simulink model "h175_model_cathode_Harness_HCTRL"  (R2023a)
settings: Solver=VariableStepAuto  StartTime=0.0  StopTime=4750  RelTol=1e-2
InitFcn:
  | run("cathode_subsystem_parameters.m")
undefined symbols (not defined in the file or in its folder): AIRCL_STATE, AIRCL_STATE_SAFETY, CSEP_STATE, CSEP_STATE_SAFETY, CSTOBLV_STATE_SAFETY, EAC_STATE, EAC_STATE_SAFETY, init_Parameters, sigbuilder_block, struct_OMM_Set, struct_Sensors
libraries: simulink x7, fl_lib x6, nesl_utility x6
settings Model: Creator=adrian.taveras  LastModifiedBy=adrian.taveras
settings SolverCC: MaxConsecutiveMinStep=20  ZeroCrossAlgorithm=Adaptive  DecoupledContinuousIntegration=on
settings DataIOCC: Refine=2
settings OptimizationCC: ReuseModelBlockBuffer=off
settings DebuggingCC: IgnoredZcDiagnostic=none
settings SimscapeCC: SimscapeLogType=all

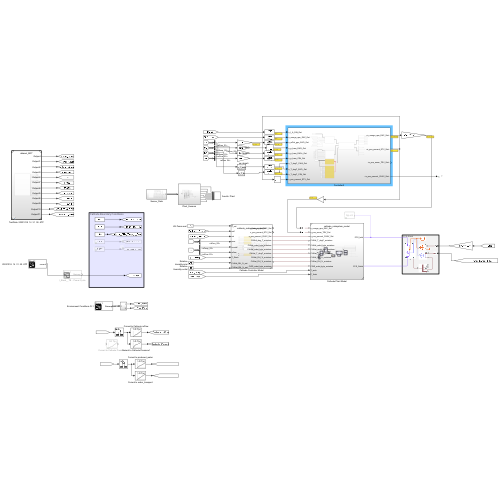
[thumbnail: Simulink's stored preview of the top-level diagram]
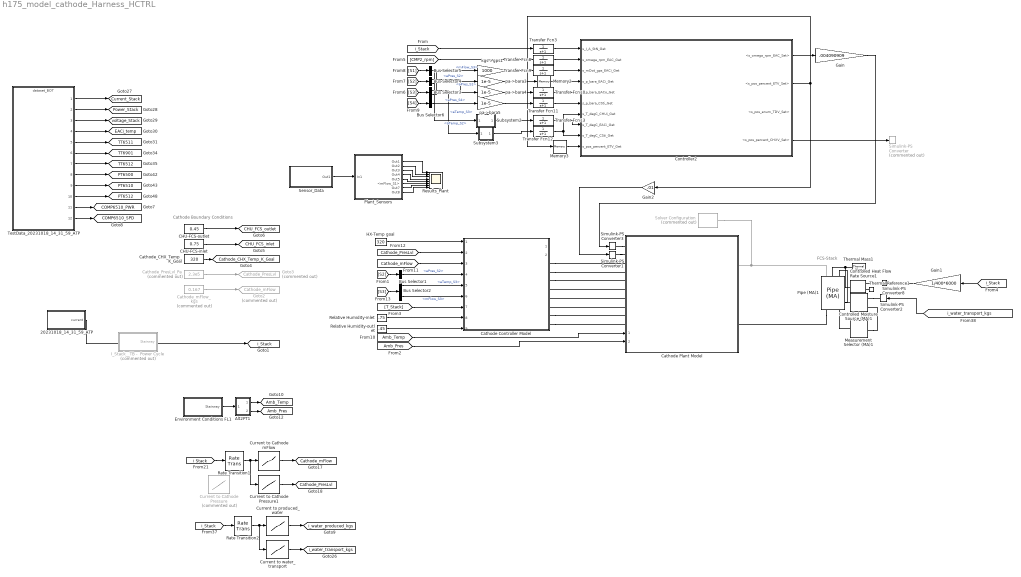
== system h175_model_cathode_Harness_HCTRL ==
  note: Cathode Boundary Conditions
  note: FCS-Stack
  20231018_14_31_59_ATP : Subsystem  Tag=STV Subsys  LoadFcn=sigbuilder_block('load');  StartFcn=sigbuilder_block('start');  StopFcn=sigbuilder_block('stop');  ClipboardFcn=sigbuilder_block('clipboard');  mask(Sigbuilder block){tuvar=[0:10]}
      mask help: Simulink:masks:SigbuilderBlock_MD
      mask init:
      | if ~strcmp(get_param(bdroot(gcbh),'SimulationStatus'),'stopped') tuvar = sigbuilder_block('maskInit'); end
      settings: CopyFcn=sigbuilder_block('copy');  DeleteFcn=sigbuilder_block('delete');  ModelCloseFcn=sigbuilder_block('modelClose');  PreSaveFcn=sigbuilder_block('preSave');  PauseFcn=sigbuilder_block('pause');  ContinueFcn=sigbuilder_block('continue');  NameChangeFcn=sigbuilder_block('namechange');  OpenFcn=sigbuilder_block('open',[725.25 330.75 938.25 556.5 ]);  CloseFcn=sigbuilder_block('close');
      mask Display: plot(0, 0, 100, 100,[2, 2, 32, 32, 2], [68, 8, 8, 68, 68],[32, 2], [38, 38], [32, 19, 2],[53, 60, 44], [32, 17, 17, 2],[16, 16, 31, 31]);txt = getActiveGroup(gcbh);text(2, 100, txt,'verticalAlignment', 'top');
  Alt2PT1 : Subsystem
  Bus Selector1 : BusSelector  OutputSignals=aPres_S2
  Bus Selector2 : BusSelector  OutputSignals=aTemp_S3,mFlow_S3
  Bus Selector3 : BusSelector  OutputSignals=aTemp_S3,mFlow_S3
  Bus Selector4 : BusSelector  OutputSignals=aPres_S2,aTemp_S2
  Bus Selector5 : BusSelector  OutputSignals=aPres_S1
  Bus Selector6 : BusSelector  OutputSignals=aPres_S4
  CHU-FCS-inlet : Constant  Value=0.75
  CHU-FCS-outlet : Constant  Value=0.45
  Cathode Controller Model : Subsystem  ReferencedSubsystem=cathode_subsystem_controller
      settings: PortSchema="{\"entries\":[{\"content\":{\"sides\":[{\"content\":{\"connectorIds\":[\"Out1\",\"Out2\",\"LConn1\",\"LConn2\",\"LConn3\",\"LConn4\",\"LConn5\",\"LConn6\",\"LConn7\",\"LConn8\"]},\"type\":\"ConnectorPlacement.EquallySpacedRectSide\",\"uuid\":\"fec6d33c-3ad3-4174-acdc-3a3b9e5715f4\"},{\"content\":{\"connectorIds\":[\"In1\",\"In2\",\"In3\",\"In4\",\"In5\",\"In6\",\"In7\",\"In8\",\"In9\"],\"side\":\"RIGHT\"},\"type\":\"ConnectorPlacement.EquallySpacedRectSide\",\"uuid\":\"4aee90de-c0ab-447d-83f7-53a254285efe\"},{\"content\":{\"side\":\"TOP\"},\"type\":\"ConnectorPlacement.EquallySpacedRectSide\",\"uuid\":\"94b2adb1-5e3a-4413-84ea-fe1e13b8a59d\"}]},\"type\":\"ConnectorPlacement.EquallySpacedConnector\",\"uuid\":\"aca8449a-2e64-4d0b-80a0-10fe30b1ea20\"}],\"packageUris\":[\"http://schema.mathworks.com/mf0/Connector/R2020b\"],\"version\":\"1.0\"}"
  Cathode Plant Model : Subsystem  ReferencedSubsystem=cathode_subsystem_model
      settings: PortSchema="{\"entries\":[{\"content\":{\"sides\":[{\"content\":{\"connectorIds\":[\"LConn10\",\"LConn9\",\"LConn1\",\"LConn2\",\"LConn3\",\"LConn4\",\"LConn5\",\"LConn6\",\"LConn7\",\"LConn8\",\"In1\",\"In2\"]},\"type\":\"ConnectorPlacement.EquallySpacedRectSide\",\"uuid\":\"e3b30cb5-20d3-4977-927f-9fea068a9234\"},{\"content\":{\"connectorIds\":[\"RConn1\",\"RConn2\"],\"side\":\"RIGHT\"},\"type\":\"ConnectorPlacement.EquallySpacedRectSide\",\"uuid\":\"2d547627-9665-492a-afa4-fcc16b1173a1\"},{\"content\":{\"side\":\"TOP\"},\"type\":\"ConnectorPlacement.EquallySpacedRectSide\",\"uuid\":\"4ee6a80a-af1f-40b1-aa59-916ec7fe1294\"}]},\"type\":\"ConnectorPlacement.EquallySpacedConnector\",\"uuid\":\"0d82e4d1-cc18-4647-90fc-0df577891cdc\"}],\"packageUris\":[\"http://schema.mathworks.com/mf0/Connector/R2020b\"],\"version\":\"1.0\"}"
  Cathode_CHX_Temp_K_Goal : Constant  Value=320
  Cathode_PresLvl_Pa : Constant  Commented=on  Value=2.3e5
  Cathode_mFlow_kgs : Constant  Commented=on  Value=0.167
  Controlled Heat Flow Rate Source1 : fl_lib/Thermal/Thermal Sources/Controlled Heat Flow Rate Source
  Controlled Moisture Source (MA)1 : fl_lib/Moist Air/Sources/Moisture & Trace Gas Sources/Controlled Moisture Source (MA)  moisture_source_spec=foundation.enum.moisture_source_spec.vapor  Phi_S_specify=off  Phi_S_priority=None  Phi_S=0 kW  Phi_S_nominal_specify=off  Phi_S_nominal_unit=kW  Phi_S_nominal_value=1  mdot_w_S_specify=off  mdot_w_S_priority=None  mdot_w_S=0 kg/s  mdot_w_S_nominal_specify=off  mdot_w_S_nominal_unit=kg/s  mdot_w_S_nominal_value=1
      settings: InternalSimscapePortConfiguration="{\"Bottom\":[],\"Left\":[{\"id\":\"S\",\"label\":\"S\",\"type\":\"foundation.moist_air.moist_air_source\"}],\"Right\":[{\"id\":\"M\",\"label\":\"M\",\"type\":\"input\"},{\"id\":\"T\",\"label\":\"T\",\"type\":\"input\"}],\"Top\":[]}"
  Controller2 : Subsystem
  Current to Cathode Pressure : Lookup_n-D  Commented=on  NumberOfTableDimensions=1  BreakpointsForDimension1=[0;50;100;150;200;250;300;350;400;510;600]  Table=[101330;110000;115000;125000;130000;140000;150000;165000;180000;200000;230000]  InternalRulePriority=Speed  RndMeth=Simplest
  Current to Cathode Pressure1 : Lookup_n-D  NumberOfTableDimensions=1  BreakpointsForDimension1=[0;50;100;150;200;250;300;350;400;510;600]  Table=[101330;140000;150000;175000;185000;195000;202500;210000;220000;235000;250000]  InternalRulePriority=Speed  RndMeth=Simplest
  Current to Cathode mFlow : Lookup_n-D  NumberOfTableDimensions=1  BreakpointsForDimension1=[0;50;100;150;200;250;300;350;400;510;600]  Table=[0;0.01;0.0225;0.035;0.045;0.055;0.068;0.0825;0.1;0.135;0.167]  InternalRulePriority=Speed  RndMeth=Simplest
  Current to produced_water : Lookup_n-D  NumberOfTableDimensions=1  BreakpointsForDimension1=[0;100;200;400;600]  Table=[0;6.491e-6;1.132e-5;1.762e-5;2.762e-5]  InternalRulePriority=Speed  RndMeth=Simplest
  Current to water_transport : Lookup_n-D  NumberOfTableDimensions=1  BreakpointsForDimension1=[0;100;200;400;600]  Table=[0;4.247e-3;8.494e-3;1.697e-2;2.548e-2]  InternalRulePriority=Speed  RndMeth=Simplest
  Environment Conditions FL1 : Subsystem  Tag=STV Subsys  LoadFcn=sigbuilder_block('load');  StartFcn=sigbuilder_block('start');  StopFcn=sigbuilder_block('stop');  ClipboardFcn=sigbuilder_block('clipboard');  mask(Sigbuilder block){tuvar=[0:10]}
      mask help: Simulink:masks:SigbuilderBlock_MD
      mask init:
      | if ~strcmp(get_param(bdroot(gcbh),'SimulationStatus'),'stopped') tuvar = sigbuilder_block('maskInit'); end
      settings: CopyFcn=sigbuilder_block('copy');  DeleteFcn=sigbuilder_block('delete');  ModelCloseFcn=sigbuilder_block('modelClose');  PreSaveFcn=sigbuilder_block('preSave');  PauseFcn=sigbuilder_block('pause');  ContinueFcn=sigbuilder_block('continue');  NameChangeFcn=sigbuilder_block('namechange');  OpenFcn=sigbuilder_block('open',[6 30 1908 951.75 ]);  CloseFcn=sigbuilder_block('close');
      mask Display: plot(0, 0, 100, 100,[2, 2, 32, 32, 2], [68, 8, 8, 68, 68],[32, 2], [38, 38], [32, 19, 2],[53, 60, 44], [32, 17, 17, 2],[16, 16, 31, 31]);txt = getActiveGroup(gcbh);text(2, 100, txt,'verticalAlignment', 'top');
  Gain : Gain  Gain=.004090909
  Gain1 : Gain  Gain=1/400*6000
  Gain2 : Gain  Gain=.01
  Goto2 : Goto  Commented=on  GotoTag=Cathode_mFlow  TagVisibility=global
  Goto3 : Goto  Commented=on  GotoTag=Cathode_PresLvl  TagVisibility=global
  HX-Temp goal : Constant  Value=320
  I_Stack__TB -  Power Cycle : Subsystem  Tag=STV Subsys  Commented=on  LoadFcn=sigbuilder_block('load');  StartFcn=sigbuilder_block('start');  StopFcn=sigbuilder_block('stop');  ClipboardFcn=sigbuilder_block('clipboard');  mask(Sigbuilder block){tuvar=[0:10]}
      mask help: Simulink:masks:SigbuilderBlock_MD
      mask init:
      | if ~strcmp(get_param(bdroot(gcbh),'SimulationStatus'),'stopped') tuvar = sigbuilder_block('maskInit'); end
      settings: CopyFcn=sigbuilder_block('copy');  DeleteFcn=sigbuilder_block('delete');  ModelCloseFcn=sigbuilder_block('modelClose');  PreSaveFcn=sigbuilder_block('preSave');  PauseFcn=sigbuilder_block('pause');  ContinueFcn=sigbuilder_block('continue');  NameChangeFcn=sigbuilder_block('namechange');  OpenFcn=sigbuilder_block('open',[329.4 141 551.4 321 ]);  CloseFcn=sigbuilder_block('close');
      mask Display: plot(0, 0, 100, 100,[2, 2, 32, 32, 2], [68, 8, 8, 68, 68],[32, 2], [38, 38], [32, 19, 2],[53, 60, 44], [32, 17, 17, 2],[16, 16, 31, 31]);txt = getActiveGroup(gcbh);text(2, 100, txt,'verticalAlignment', 'top');
  Measurement Selector (MA)1 : fl_lib/Moist Air/Sensors/Measurement Selector (MA)  moisture_spec=foundation.enum.moisture_spec.relative_humidity  trace_gas_spec=foundation.enum.trace_gas_spec.mole_fraction
  Memory2 : Memory  InitialCondition=1
  Memory3 : Memory  InitialCondition=1
  Pipe (MA)1 : fl_lib/Moist Air/Elements/Pipe (MA)  length=1 m  area=1 m^2  Dh=.1 m  length_add=.1 m  roughness=15e-6 m  Re_lam=2000  Re_tur=4000  shape_factor=1  Nu_lam=3.66  wall_condensation=simscape.enum.onoff.on  RH_ws=1  time_constant=1e-3 s  moisture_trace_gas_source=foundation.enum.moisture_trace_gas_source.controlled  moisture_source_spec=foundation.enum.moisture_source_spec.vapor  moisture_mass_flow=0 kg/s  moisture_temperature_spec=foundation.enum.temperature_spec.atmospheric  moisture_temperature=293.15 K  trace_gas_mass_flow=0 kg/s  trace_gas_temperature_spec=foundation.enum.temperature_spec.atmospheric  trace_gas_temperature=293.15 K  p_I_specify=off  p_I_priority=High  p_I=0.101325 MPa  p_I_nominal_specify=off  p_I_nominal_unit=MPa  p_I_nominal_value=1  T_I_specify=off  T_I_priority=High  T_I=293.15 K  T_I_nominal_specify=off  T_I_nominal_unit=K  T_I_nominal_value=1  RH_I_specify=off  RH_I_priority=High  RH_I=0  RH_I_nominal_specify=off  RH_I_nominal_unit=1  RH_I_nominal_value=1  x_w_I_specify=off  x_w_I_priority=None  x_w_I=0  x_w_I_nominal_specify=off  x_w_I_nominal_unit=1  x_w_I_nominal_value=1  y_w_I_specify=off  y_w_I_priority=None  y_w_I=0  y_w_I_nominal_specify=off  y_w_I_nominal_unit=1  y_w_I_nominal_value=1  HR_I_specify=off  HR_I_priority=None  HR_I=0  HR_I_nominal_specify=off  HR_I_nominal_unit=1  HR_I_nominal_value=1  x_g_I_specify=off  x_g_I_priority=High  x_g_I=0  x_g_I_nominal_specify=off  x_g_I_nominal_unit=1  x_g_I_nominal_value=1  y_g_I_specify=off  y_g_I_priority=None  y_g_I=0  y_g_I_nominal_specify=off  y_g_I_nominal_unit=1  y_g_I_nominal_value=1
      settings: InternalSimscapePortConfiguration="{\"Bottom\":[],\"Left\":[{\"id\":\"A\",\"label\":\"A\",\"type\":\"foundation.moist_air.moist_air\"},{\"id\":\"H\",\"label\":\"H\",\"type\":\"foundation.thermal.thermal\"},{\"id\":\"S\",\"label\":\"S\",\"type\":\"foundation.moist_air.moist_air_source\"}],\"Right\":[{\"id\":\"B\",\"label\":\"B\",\"type\":\"foundation.moist_air.moist_air\"},{\"id\":\"W\",\"label\":\"W\",\"type\":\"output\"},{\"id\":\"F\",\"label\":\"F\",\"type\":\"output\"}],\"Top\":[]}"
  Plant_Sensors : Subsystem
  Rate Transition1 : RateTransition
  Rate Transition2 : RateTransition
  Relative Humidity-inlet : Constant  Value=.75
  Relative Humidity-outlet : Constant  Value=.45
  Results_Plant : Scope  NumInputPorts=8
  Sensor_Data : Subsystem
  Simulink-PS Converter : nesl_utility/Simulink-PS Converter  Commented=on  PhysicalDomain=network_engine_domain  SubClassName=ps_input  LeftPortType=input  RightPortType=output  PseudoPeriodic=off  Frequencies=[]  NoiseDistribution=none  NoiseParameters=[]  Unit=1  AffineConversion=off  FilteringAndDerivatives=provide  SimscapeFilterOrder=1  InputFilterTimeConstant=0.001  UdotUserProvided=0
  Simulink-PS Converter1 : nesl_utility/Simulink-PS Converter  PhysicalDomain=network_engine_domain  SubClassName=ps_input  LeftPortType=input  RightPortType=output  PseudoPeriodic=off  Frequencies=[]  NoiseDistribution=none  NoiseParameters=[]  Unit=1  AffineConversion=off  FilteringAndDerivatives=provide  SimscapeFilterOrder=1  InputFilterTimeConstant=0.001  UdotUserProvided=0
  Simulink-PS Converter2 : nesl_utility/Simulink-PS Converter  PhysicalDomain=network_engine_domain  SubClassName=ps_input  LeftPortType=input  RightPortType=output  PseudoPeriodic=off  Frequencies=[]  NoiseDistribution=none  NoiseParameters=[]  Unit=1  AffineConversion=off  FilteringAndDerivatives=provide  SimscapeFilterOrder=1  InputFilterTimeConstant=0.001  UdotUserProvided=0
  Simulink-PS Converter3 : nesl_utility/Simulink-PS Converter  PhysicalDomain=network_engine_domain  SubClassName=ps_input  LeftPortType=input  RightPortType=output  PseudoPeriodic=off  Frequencies=[]  NoiseDistribution=none  NoiseParameters=[]  Unit=1  AffineConversion=off  FilteringAndDerivatives=provide  SimscapeFilterOrder=1  InputFilterTimeConstant=0.001  UdotUserProvided=0
  Simulink-PS Converter8 : nesl_utility/Simulink-PS Converter  PhysicalDomain=network_engine_domain  SubClassName=ps_input  LeftPortType=input  RightPortType=output  PseudoPeriodic=off  Frequencies=[]  NoiseDistribution=none  NoiseParameters=[]  Unit=W  AffineConversion=off  FilteringAndDerivatives=provide  SimscapeFilterOrder=1  InputFilterTimeConstant=0.001  UdotUserProvided=0
  Solver Configuration : nesl_utility/Solver Configuration  Commented=on  PhysicalDomain=network_engine_domain  SubClassName=solver  LeftPortType=input  RightPortType=generic  Tones=[]  Harmonics=[]  SimulateNoise=off  Profile=off  UseLocalSampling=off  EnableSwitchedLinearOptims=on  FrequencyDomain=off  UseCCode=off  RelTol=0.001  AbsTol=0.001  MinStep=1e-09  ToWorkspace=off  RevertToSquareIcSolve=off  NumHomotopyIterations=100  PhasorMode=off  PhasorModeNumHarmonics=1  ConsistencySolver=NEWTON_XTOL_AFTER_FTOL  IndexReductionMethod=DerivativeReplacement  DoDC=off  ResidualTolerance=1e-09  ConsistencyTolSource=GLOBAL  ConsistencyAbsTol=0.001  ConsistencyRelTol=0.001  ConsistencyTolFactor=0.001  UseLocalSolver=off  LocalSolverChoice=NE_BACKWARD_EULER_ADVANCER  ResolveIndetEquations=on  FunctionEvalNumThread=1  LocalSolverSampleTime=0.001  DoFixedCost=off  MaxNonlinIter=3  MaxModeIter=2  ComputeImpulses=off  ImpulseIterations=2  LinearAlgebra=auto  LinearAlgebraNumThread=0  EquationFormulation=NE_TIME_EF  DelaysMemoryBudget=1024  AutomaticFiltering=on  FilteringTimeConstant=0.001  PartitionStorageMethod=AS_NEEDED  PartitionMemoryBudget=1024  PartitionMethod=ROBUST
  Subsystem2 : Subsystem
  Subsystem3 : Subsystem
  TestData_20231018_14_31_59_ATP : ModelReference  ModelNameDialog=dataset_BOT.slx  SimulationMode=Normal  ModelReferenceVersion=1.7
  Thermal Mass1 : fl_lib/Thermal/Thermal Elements/Thermal Mass  mass_type=foundation.enum.constant_variable.constant  mass=10 kg  sp_heat=447 J/(K*kg)  mass_min=1e-6 kg  num_ports=foundation.enum.numPorts2.one  m_specify=off  m_priority=High  m=1 kg  m_nominal_specify=off  m_nominal_unit=kg  m_nominal_value=1  T_specify=off  T_priority=High  T=300 K  T_nominal_specify=off  T_nominal_unit=K  T_nominal_value=1  Q_specify=off  Q_priority=None  Q=0 W  Q_nominal_specify=off  Q_nominal_unit=W  Q_nominal_value=1
  Thermal Reference1 : fl_lib/Thermal/Thermal Elements/Thermal Reference
  Transfer Fcn{3,8..13} (7 alike) : TransferFcn  Denominator=[1 1]
  kgs->gps1 : Gain  Gain=1000
  pa->bara3 : Gain  Gain=1e-5
  pa->bara4 : Gain  Gain=1e-5
  pa->bara5 : Gain  Gain=1e-5
  tag scope: Amb_Pres=global, Amb_Temp=global, CHU_FCS_inlet=global, CHU_FCS_outlet=global, COMP6510_PWR=global, COMP6510_SPD=global, Cathode_CHX_Temp_K_Goal=global, Cathode_PresLvl=global, Cathode_mFlow=global, Current_Stack=global, EACi_temp=global, PT6500=global, PT6510=global, PT6512=global, Power_Stack=global, TT6511=global, TT6512=global, TT6901=global, i_Stack=global, i_water_produced_kgs=global, i_water_transport_kgs=global, voltage_Stack=global
  wires:
  Plant_Sensors/1(Out1) -> Results_Plant/1
  Plant_Sensors/2(Out2) -> Results_Plant/2
  Plant_Sensors/3(Out3) -> Results_Plant/3
  Plant_Sensors/4(Out4) -> Results_Plant/4
  Plant_Sensors/5(Out5) -> Results_Plant/5
  Plant_Sensors/6(<mFlow_S1>) -> Results_Plant/6
  Plant_Sensors/7(Out7) -> Results_Plant/7
  Plant_Sensors/8(Out8) -> Results_Plant/8
  Cathode_PresLvl_Pa/1 -> Goto3/1
  Cathode_mFlow_kgs/1 -> Goto2/1
  CHU-FCS-outlet/1 -> [CHU_FCS_outlet]
  CHU-FCS-inlet/1 -> [CHU_FCS_inlet]
  Cathode_CHX_Temp_K_Goal/1 -> [Cathode_CHX_Temp_K_Goal]
  Alt2PT1/2(Out2) -> [Amb_Pres]
  Environment Conditions FL1/1(Stairway) -> Alt2PT1/1(In1)
  Alt2PT1/1(Out1) -> [Amb_Temp]
  Current to Cathode mFlow/1 -> [Cathode_mFlow]
  Rate Transition1/1 -> Current to Cathode Pressure1/1, Current to Cathode mFlow/1
  Current to Cathode Pressure1/1 -> [Cathode_PresLvl]
  [i_Stack] -> Rate Transition1/1
  [Amb_Temp] -> Cathode Plant Model/1
  [S2] -> Bus Selector1/1
  [Cathode_mFlow] -> Cathode Controller Model/3
  Relative Humidity-inlet/1 -> Cathode Controller Model/8
  Relative Humidity-outlet/1 -> Cathode Controller Model/9
  [T_Stack] -> Cathode Controller Model/7
  Bus Selector1/1 -> Cathode Controller Model/4  "<aPres_S2>"
  [Amb_Pres] -> Cathode Plant Model/2
  Bus Selector2/1 -> Cathode Controller Model/5  "<aTemp_S3>"
  HX-Temp goal/1 -> Cathode Controller Model/1
  [S3] -> Bus Selector2/1
  Bus Selector2/2 -> Cathode Controller Model/6  "<mFlow_S3>"
  [Cathode_PresLvl] -> Cathode Controller Model/2
  20231018_14_31_59_ATP/1(current) -> [i_Stack]
  Sensor_Data/1(Out1) -> Plant_Sensors/1(In1)
  Gain1/1 -> Simulink-PS Converter8/1
  [i_Stack] -> Gain1/1
  [i_water_transport_kgs] -> Simulink-PS Converter2/1
  TestData_20231018_14_31_59_ATP/1 -> [Current_Stack]
  TestData_20231018_14_31_59_ATP/2 -> [Power_Stack]
  TestData_20231018_14_31_59_ATP/3 -> [voltage_Stack]
  TestData_20231018_14_31_59_ATP/4 -> [EACi_temp]
  TestData_20231018_14_31_59_ATP/5 -> [TT6511]
  TestData_20231018_14_31_59_ATP/6 -> [TT6901]
  TestData_20231018_14_31_59_ATP/7 -> [TT6512]
  TestData_20231018_14_31_59_ATP/11 -> [COMP6510_PWR]
  TestData_20231018_14_31_59_ATP/12 -> [COMP6510_SPD]
  TestData_20231018_14_31_59_ATP/10 -> [PT6512]
  TestData_20231018_14_31_59_ATP/9 -> [PT6510]
  TestData_20231018_14_31_59_ATP/8 -> [PT6500]
  Bus Selector3/1 -> Subsystem3/1(s_T_degC_EACi_Get)  "<aTemp_S3>"
  Transfer Fcn10/1 -> Controller2/5(s_p_bara_EACo_Get)
  Subsystem2/1(Out1) -> Transfer Fcn13/1
  Bus Selector6/1 -> pa->bara5/1  "<aPres_S4>"
  Transfer Fcn3/1 -> Controller2/1(s_I_A_StN_Get)
  Bus Selector4/1 -> pa->bara4/1  "<aPres_S2>"
  [S2] -> Bus Selector4/1
  pa->bara3/1 -> Memory2/1
  Transfer Fcn13/1 -> Controller2/8(s_T_degC_EACi_Get)
  Bus Selector5/1 -> pa->bara3/1  "<aPres_S1>"
  [S1] -> Bus Selector5/1
  pa->bara5/1 -> Transfer Fcn11/1
  kgs->gps1/1 -> Transfer Fcn9/1
  Subsystem3/1(Out1) -> Transfer Fcn12/1
  Memory2/1 -> Controller2/4(s_p_bara_EACi_Get)
  Transfer Fcn8/1 -> Controller2/2(s_omega_rpm_EAC_Get)
  pa->bara4/1 -> Transfer Fcn10/1
  Bus Selector4/2 -> Subsystem2/1(s_T_degC_EACi_Get)  "<aTemp_S2>"
  Controller2/4(<s_pos_percent_CHXV_Set>) -> Simulink-PS Converter/1
  [S4] -> Bus Selector6/1
  [CMP2_rpm] -> Transfer Fcn8/1
  Memory3/1 -> Controller2/10(s_pos_percent_ETV_Get)
  [i_Stack] -> Transfer Fcn3/1
  [S3] -> Bus Selector3/1
  Transfer Fcn11/1 -> Controller2/6(s_p_bara_CSti_Get)
  Bus Selector3/2 -> kgs->gps1/1  "<mFlow_S3>"
  Transfer Fcn12/1 -> Controller2/9(s_T_degC_CSti_Get), Controller2/7(s_T_degC_CHUi_Get)
  Transfer Fcn9/1 -> Controller2/3(s_mDot_gps_EACi_Get)
  Controller2/1(<s_omega_rpm_EAC_Set>) -> Gain/1
  Controller2/2(<s_pos_percent_ETV_Set>) -> Gain2/1, Memory3/1
  Rate Transition2/1 -> Current to water_transport/1, Current to produced_water/1
  [i_Stack] -> Rate Transition2/1
  Current to water_transport/1 -> [i_water_transport_kgs]
  Current to produced_water/1 -> [i_water_produced_kgs]
  Gain2/1 -> Simulink-PS Converter1/1
  Gain/1 -> Simulink-PS Converter3/1
  connections:
  Solver Configuration/RConn1 -- Pipe (MA)1/LConn1 -- Cathode Plant Model/RConn1
  Cathode Controller Model/LConn3 -- Cathode Plant Model/LConn3
  Cathode Controller Model/LConn1 -- Cathode Plant Model/LConn1
  Cathode Plant Model/LConn5 -- Cathode Controller Model/LConn5
  Cathode Plant Model/LConn6 -- Cathode Controller Model/LConn6
  Cathode Plant Model/LConn4 -- Cathode Controller Model/LConn4
  Cathode Controller Model/LConn2 -- Cathode Plant Model/LConn2
  Cathode Controller Model/LConn7 -- Cathode Plant Model/LConn7
  Cathode Controller Model/LConn8 -- Cathode Plant Model/LConn8
  Thermal Mass1/LConn1 -- Controlled Heat Flow Rate Source1/LConn1 -- Pipe (MA)1/LConn2
  Measurement Selector (MA)1/RConn2 -- Controlled Moisture Source (MA)1/RConn2
  Thermal Reference1/LConn1 -- Controlled Heat Flow Rate Source1/RConn2
  Pipe (MA)1/RConn3 -- Measurement Selector (MA)1/LConn1
  Pipe (MA)1/RConn1 -- Cathode Plant Model/RConn2
  Controlled Moisture Source (MA)1/LConn1 -- Pipe (MA)1/LConn3
  Simulink-PS Converter8/RConn1 -- Controlled Heat Flow Rate Source1/RConn1
  Controlled Moisture Source (MA)1/RConn1 -- Simulink-PS Converter2/RConn1
  Simulink-PS Converter1/RConn1 -- Cathode Plant Model/LConn9
  Simulink-PS Converter3/RConn1 -- Cathode Plant Model/LConn10

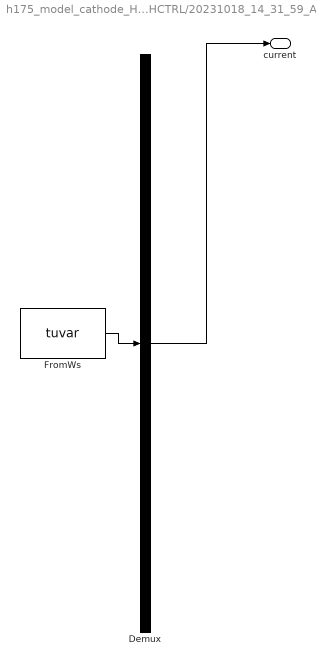
== system h175_model_cathode_Harness_HCTRL/20231018_14_31_59_ATP ==
  Demux : Demux  Tag=STV Demux  Outputs=1
      settings: DisplayOption=none
  FromWs : FromWorkspace  Tag=STV FromWs  VariableName=tuvar
      SigBuilderData=|
      | common.afterFinalStr = 'Extrapolate'
      | common.sampleTime = 0
      | dataSet.timeRange = [0 4735]
      | dataSet.name = 'Sheet1'
      | sbobj.Groups.Name = 'Sheet1'
      | sbobj.Groups.Signals.Name = 'current'
      | sbobj.Groups.Signals.XData = [0 710 730 830 850 1000 1020 1080 1100 1200 1230 1260 1270 1320 1340 1390 1405 1455 1475 1525 1565 3990 4000 4030 4090 4130 4245 4270 4345 4355 4385 4395 4735]
      | sbobj.Groups.Signals.YData = [5 5 45 45 100 100 200 200 300 300 45 45 50 50 200 200 300 300 100 100 420 420 340 420 260 340 340 50 50 45 45 5 5]
      | sbobj.Groups.TimeRange = [0 4735]
  current : Outport  Tag=STV Outport
  wires:
  Demux/1 -> current/1
  FromWs/1 -> Demux/1

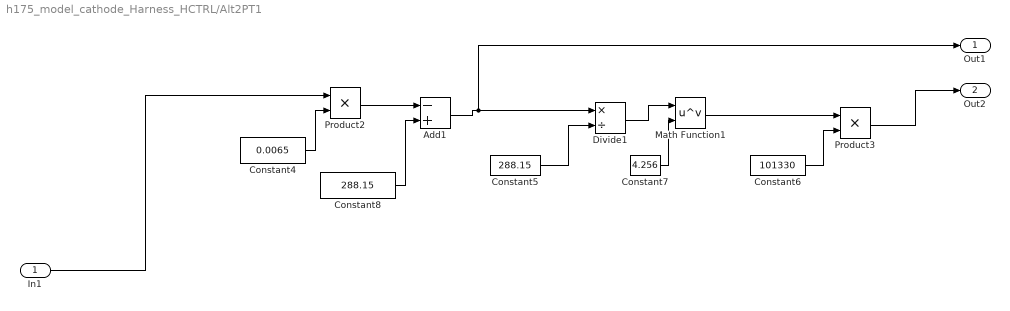
== system h175_model_cathode_Harness_HCTRL/Alt2PT1 ==
  In1 : Inport
  Add1 : Sum  Inputs=-+
  Constant4 : Constant  Value=0.0065
  Constant5 : Constant  Value=288.15
  Constant6 : Constant  Value=101330
  Constant7 : Constant  Value=4.256
  Constant8 : Constant  Value=288.15
  Divide1 : Product  Inputs=*/
  Math Function1 : Math  Operator=pow
  Product2 : Product
  Product3 : Product
  Out1 : Outport
  Out2 : Outport  Port=2
  wires:
  Constant5/1 -> Divide1/2
  Constant8/1 -> Add1/2
  In1/1 -> Product2/1
  Add1/1 -> Out1/1, Divide1/1
  Constant4/1 -> Product2/2
  Math Function1/1 -> Product3/1
  Constant7/1 -> Math Function1/2
  Divide1/1 -> Math Function1/1
  Product2/1 -> Add1/1
  Constant6/1 -> Product3/2
  Product3/1 -> Out2/1

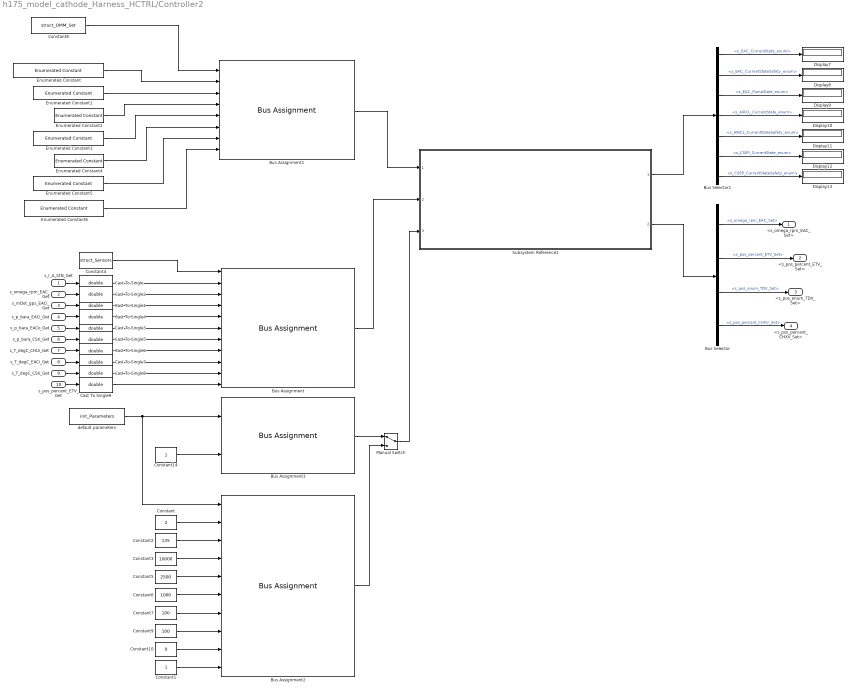
== system h175_model_cathode_Harness_HCTRL/Controller2 ==
  s_I_A_StN_Get : Inport
  s_omega_rpm_EAC_Get : Inport  Port=2
  s_mDot_gps_EACi_Get : Inport  Port=3
  s_p_bara_EACi_Get : Inport  Port=4
  s_p_bara_EACo_Get : Inport  Port=5
  s_p_bara_CSti_Get : Inport  Port=6
  s_T_degC_CHUi_Get : Inport  Port=7
  s_T_degC_EACi_Get : Inport  Port=8
  s_T_degC_CSti_Get : Inport  Port=9
  s_pos_percent_ETV_Get : Inport  Port=10
  Bus Assignment : BusAssignment  AssignedSignals=b_ElectricalSens.b_Sens_IVT.s_I_A_StN_Get,b_CathodeSens.b_EAC_SENS.s_omega_rpm_EAC_Get,b_CathodeSens.b_mdotSens_EACi.s_mDot_gps_EACi_Get,b_CathodeSens.b_pSens_EACi.s_p_bara_EACi_Get,b_CathodeSens.b_pSens_EACo.s_p_bara_EACo_Get,b_CathodeSens.b_pSens_CSti.s_p_bara_CSti_Get,b_CathodeSens.b_TSens_CHUi.s_T_degC_CHUi_Get,b_CathodeSens.b_TSens_EACi.s_T_degC_EACi_Get,b_CathodeSens.b_TSens_CSti.s_T_degC_CSti_Get,b_CathodeSens.b_ETV_SENS.s_pos_percent_ETV_Get
  Bus Assignment1 : BusAssignment  AssignedSignals=b_OMM_Cathode_Set.s_EAC_StateSetREQ_enum,b_OMM_Cathode_Set.s_EAC_ForceShutdownState_enum,b_OMM_Cathode_Set.s_AIRCL_StateSetREQ_enum,b_OMM_Cathode_Set.s_AIRCL_ForceShutdownState_enum,b_OMM_Cathode_Set.s_CSEP_StateSetREQ_enum,b_OMM_Cathode_Set.s_CSEP_ForceShutdownState_enum,b_OMM_Cathode_Set.s_CStoBlV_ForceShutdownState_enum
  Bus Assignment2 : BusAssignment  AssignedSignals=b_CAT_Parameters.b_EAC_Parameters.p_EAC_ETVctrl_mode_switch,b_CAT_Parameters.b_EAC_Parameters.p_EAC_SP_ConstMassflow1_mDot_gps,b_CAT_Parameters.b_EAC_Parameters.p_Fis_EAC_pCtrl_PID_P,b_CAT_Parameters.b_EAC_Parameters.p_Fis_EAC_pCtrl_PID_I,b_CAT_Parameters.b_EAC_Parameters.p_Fis_EAC_pCtrl_PID_D,b_CAT_Parameters.b_EAC_Parameters.p_Fis_EAC_pCtrl_PID_Offset_pos_per,b_CAT_Parameters.b_EAC_Parameters.p_Fis_EAC_pCtrl_PID_UpperLim_pos_per,b_CAT_Parameters.b_EAC_Parameters.p_Fis_EAC_pCtrl_PID_LowerLim_pos_per,b_CAT_Parameters.b_EAC_Parameters.p_Fis_EAC_pCtrl_PID_Filtr_T
  Bus Assignment3 : BusAssignment  AssignedSignals=b_CAT_Parameters.b_EAC_Parameters.p_EAC_ETVctrl_mode_switch
  Bus Selector : BusSelector  OutputSignals=b_EAC_ACT.s_omega_rpm_EAC_Set,b_ETV_ACT.s_pos_percent_ETV_Set,b_TDV_ACT.s_pos_enum_TDV_Set,b_CHXV_ACT.s_pos_percent_CHXV_Set
  Bus Selector1 : BusSelector  OutputSignals=s_EAC_CurrentState_enum,s_EAC_CurrentStateSafety_enum,s_EAC_PumpState_enum,s_AIRCL_CurrentState_enum,s_AIRCL_CurrentStateSafety_enum,s_CSEP_CurrentState_enum,s_CSEP_CurrentStateSafety_enum
  Cast To Single{,1..9} (10 alike) : DataTypeConversion  OutDataTypeStr=double  SaturateOnIntegerOverflow=off  RndMeth=Floor
  Constant : Constant  Value=2  OutDataTypeStr=double
  Constant1 : Constant  OutDataTypeStr=double
  Constant10 : Constant  Value=0  OutDataTypeStr=double
  Constant14 : Constant  OutDataTypeStr=double
  Constant2 : Constant  Value=135  OutDataTypeStr=double
  Constant3 : Constant  Value=10000  OutDataTypeStr=double
  Constant4 : Constant  Value=struct_Sensors  OutDataTypeStr=Bus: Sensors
  Constant5 : Constant  Value=2500  OutDataTypeStr=double
  Constant6 : Constant  Value=1000  OutDataTypeStr=double
  Constant7 : Constant  Value=100  OutDataTypeStr=double
  Constant8 : Constant  Value=struct_OMM_Set  OutDataTypeStr=Bus: OMM_Set
  Constant9 : Constant  Value=100  OutDataTypeStr=double
  Display{7..13} (7 alike) : Display
  Enumerated Constant : simulink/Sources/Enumerated Constant  OutDataTypeStr=Enum: EAC_STATE  Value=EAC_STATE.constMassflow1  SampleTime=inf
  Enumerated Constant1 : simulink/Sources/Enumerated Constant  OutDataTypeStr=Enum: EAC_STATE_SAFETY  Value=EAC_STATE_SAFETY.Safe  SampleTime=inf
  Enumerated Constant2 : simulink/Sources/Enumerated Constant  OutDataTypeStr=Enum: AIRCL_STATE  Value=AIRCL_STATE.On  SampleTime=inf
  Enumerated Constant3 : simulink/Sources/Enumerated Constant  OutDataTypeStr=Enum: AIRCL_STATE_SAFETY  Value=AIRCL_STATE_SAFETY.Safe  SampleTime=inf
  Enumerated Constant4 : simulink/Sources/Enumerated Constant  OutDataTypeStr=Enum: CSEP_STATE  Value=CSEP_STATE.Opened  SampleTime=inf
  Enumerated Constant5 : simulink/Sources/Enumerated Constant  OutDataTypeStr=Enum: CSEP_STATE_SAFETY  Value=CSEP_STATE_SAFETY.Safe  SampleTime=inf
  Enumerated Constant6 : simulink/Sources/Enumerated Constant  OutDataTypeStr=Enum: CSTOBLV_STATE_SAFETY  Value=CSTOBLV_STATE_SAFETY.Safe  SampleTime=inf
  Manual Switch : ManualSwitch
  Subsystem Reference1 : Subsystem  ReferencedSubsystem=CathodeSubsystem
  default parameters : Constant  Value=init_Parameters  OutDataTypeStr=Bus: Parameters
  <s_omega_rpm_EAC_Set> : Outport
  <s_pos_percent_ETV_Set> : Outport  Port=2
  <s_pos_enum_TDV_Set> : Outport  Port=3
  <s_pos_percent_CHXV_Set> : Outport  Port=4
  wires:
  Constant/1 -> Bus Assignment2/2
  Bus Selector1/4 -> Display10/1  "<s_AIRCL_CurrentState_enum>"
  Enumerated Constant/1 -> Bus Assignment1/2
  Bus Assignment1/1 -> Subsystem Reference1/1
  Enumerated Constant6/1 -> Bus Assignment1/8
  Constant8/1 -> Bus Assignment1/1
  Bus Selector1/2 -> Display8/1  "<s_EAC_CurrentStateSafety_enum>"
  s_I_A_StN_Get/1 -> Cast To Single/1
  s_p_bara_EACi_Get/1 -> Cast To Single4/1
  Bus Selector1/5 -> Display11/1  "<s_AIRCL_CurrentStateSafety_enum>"
  Subsystem Reference1/2 -> Bus Selector/1
  Bus Assignment/1 -> Subsystem Reference1/2
  Enumerated Constant2/1 -> Bus Assignment1/4
  Enumerated Constant5/1 -> Bus Assignment1/7
  Enumerated Constant1/1 -> Bus Assignment1/3
  Enumerated Constant3/1 -> Bus Assignment1/5
  Enumerated Constant4/1 -> Bus Assignment1/6
  Bus Selector1/3 -> Display9/1  "<s_EAC_PumpState_enum>"
  Bus Selector1/6 -> Display12/1  "<s_CSEP_CurrentState_enum>"
  s_T_degC_CSti_Get/1 -> Cast To Single8/1
  Bus Selector1/1 -> Display7/1  "<s_EAC_CurrentState_enum>"
  s_T_degC_EACi_Get/1 -> Cast To Single7/1
  Bus Selector1/7 -> Display13/1  "<s_CSEP_CurrentStateSafety_enum>"
  Subsystem Reference1/1 -> Bus Selector1/1
  Bus Selector/3 -> <s_pos_enum_TDV_Set>/1  "<s_pos_enum_TDV_Set>"
  s_omega_rpm_EAC_Get/1 -> Cast To Single2/1
  Bus Selector/4 -> <s_pos_percent_CHXV_Set>/1  "<s_pos_percent_CHXV_Set>"
  Constant4/1 -> Bus Assignment/1
  default parameters/1 -> Bus Assignment2/1, Bus Assignment3/1
  Bus Selector/1 -> <s_omega_rpm_EAC_Set>/1  "<s_omega_rpm_EAC_Set>"
  s_mDot_gps_EACi_Get/1 -> Cast To Single1/1
  s_p_bara_EACo_Get/1 -> Cast To Single3/1
  s_p_bara_CSti_Get/1 -> Cast To Single5/1
  s_T_degC_CHUi_Get/1 -> Cast To Single6/1
  Bus Selector/2 -> <s_pos_percent_ETV_Set>/1  "<s_pos_percent_ETV_Set>"
  s_pos_percent_ETV_Get/1 -> Cast To Single9/1
  Constant2/1 -> Bus Assignment2/3
  Constant3/1 -> Bus Assignment2/4
  Constant5/1 -> Bus Assignment2/5
  Constant6/1 -> Bus Assignment2/6
  Constant9/1 -> Bus Assignment2/8
  Constant10/1 -> Bus Assignment2/9
  Constant1/1 -> Bus Assignment2/10
  Constant14/1 -> Bus Assignment3/2
  Bus Assignment3/1 -> Manual Switch/1
  Manual Switch/1 -> Subsystem Reference1/3
  Bus Assignment2/1 -> Manual Switch/2
  Constant7/1 -> Bus Assignment2/7
  Cast To Single/1 -> Bus Assignment/2
  Cast To Single7/1 -> Bus Assignment/9
  Cast To Single2/1 -> Bus Assignment/3
  Cast To Single1/1 -> Bus Assignment/4
  Cast To Single4/1 -> Bus Assignment/5
  Cast To Single3/1 -> Bus Assignment/6
  Cast To Single5/1 -> Bus Assignment/7
  Cast To Single6/1 -> Bus Assignment/8
  Cast To Single8/1 -> Bus Assignment/10
  Cast To Single9/1 -> Bus Assignment/11

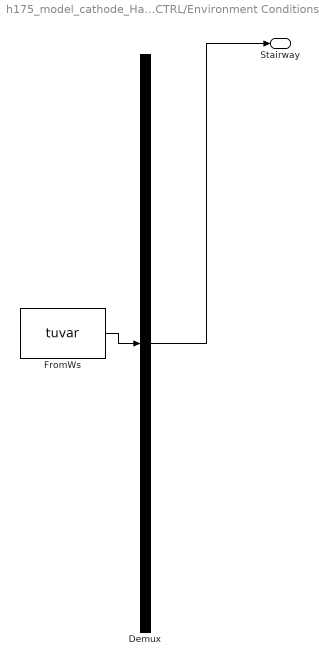
== system h175_model_cathode_Harness_HCTRL/Environment Conditions FL1 ==
  Demux : Demux  Tag=STV Demux  Outputs=1
      settings: DisplayOption=none
  FromWs : FromWorkspace  Tag=STV FromWs  VariableName=tuvar
      SigBuilderData=|
      | common.afterFinalStr = 'Extrapolate'
      | common.sampleTime = 0
      | dataSet.timeRange = [0 22226]
      | dataSet.name = 'Group 1'
      | sbobj.Groups.Name = 'Group 1'
      | sbobj.Groups.Signals.Name = 'Stairway'
      | sbobj.Groups.Signals.XData = [0 1 1.1 1.2 1.3 120 270 670 1450 7450 7510 21146 21826 22226]
      | sbobj.Groups.Signals.YData = [0 0 0 0 0 0 250 650 1100 1100 1000 1000 500 0]
      | sbobj.Groups.TimeRange = [0 22226]
  Stairway : Outport  Tag=STV Outport
  wires:
  Demux/1 -> Stairway/1
  FromWs/1 -> Demux/1

== system h175_model_cathode_Harness_HCTRL/I_Stack__TB -  Power Cycle ==
  Demux : Demux  Tag=STV Demux  Outputs=1
      settings: DisplayOption=none
  FromWs : FromWorkspace  Tag=STV FromWs  VariableName=tuvar
      SigBuilderData=|
      | common.afterFinalStr = 'Extrapolate'
      | common.sampleTime = 0
      | dataSet.timeRange = [0 600]
      | dataSet.name = 'Group 1'
      | sbobj.Groups.Name = 'Group 1'
      | sbobj.Groups.Signals.Name = 'Stairway'
      | sbobj.Groups.Signals.XData = [0 180 190 250 260 320 330 390 410 460 470 530 540 600]
      | sbobj.Groups.Signals.YData = [100 100 200 200 400 400 600 600 300 300 200 200 100 100]
      | sbobj.Groups.TimeRange = [0 600]
  Stairway : Outport  Tag=STV Outport
  wires:
  Demux/1 -> Stairway/1
  FromWs/1 -> Demux/1

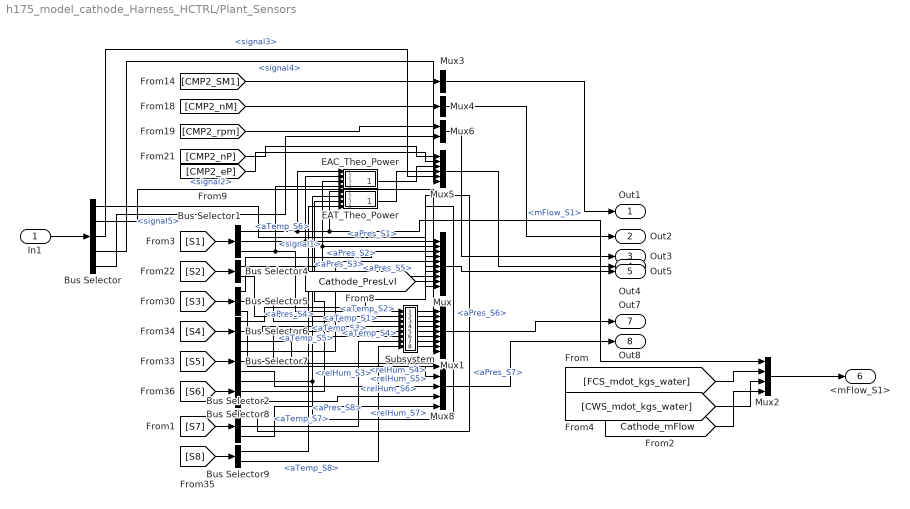
== system h175_model_cathode_Harness_HCTRL/Plant_Sensors ==
  In1 : Inport
  Bus Selector : BusSelector  OutputSignals=signal1,signal2,signal3,signal4,signal5
  Bus Selector1 : BusSelector  OutputSignals=mFlow_S1,aPres_S1,aTemp_S1
  Bus Selector2 : BusSelector  OutputSignals=aPres_S7,aTemp_S7,relHum_S7
  Bus Selector4 : BusSelector  OutputSignals=aPres_S2,aTemp_S2
  Bus Selector5 : BusSelector  OutputSignals=aPres_S3,aTemp_S3,relHum_S3
  Bus Selector6 : BusSelector  OutputSignals=aPres_S4,aTemp_S4,relHum_S4
  Bus Selector7 : BusSelector  OutputSignals=aPres_S5,aTemp_S5,relHum_S5
  Bus Selector8 : BusSelector  OutputSignals=aPres_S6,aTemp_S6,relHum_S6
  Bus Selector9 : BusSelector  OutputSignals=aPres_S8,aTemp_S8
  EAC_Theo_Power : Subsystem
  EAT_Theo_Power : Subsystem
  Mux : Mux  Inputs=10
  Mux1 : Mux  Inputs=9
  Mux2 : Mux
  Mux3 : Mux  Inputs=1
  Mux4 : Mux  Inputs=1
  Mux5 : Mux  Inputs=6
  Mux6 : Mux  Inputs=2
  Mux8 : Mux  Inputs=5
  Subsystem : Subsystem
  Out1 : Outport
  Out2 : Outport  Port=2
  Out3 : Outport  Port=3
  Out4 : Outport  Port=4
  Out5 : Outport  Port=5
  <mFlow_S1> : Outport  Port=6
  Out7 : Outport  Port=7
  Out8 : Outport  Port=8
  wires:
  [CMP2_eP] -> Mux5/2
  [CMP2_nP] -> Mux5/1
  Mux3/1 -> Out1/1
  [S8] -> Bus Selector9/1
  [CMP2_SM1] -> Mux3/1
  Bus Selector7/3 -> Mux8/3  "<relHum_S5>"
  Bus Selector9/1 -> EAT_Theo_Power/4(<aPres_S7>), Mux/8  "<aPres_S8>"
  Bus Selector4/1 -> EAC_Theo_Power/3(<aPres_S2>), Mux/2  "<aPres_S2>"
  [CMP2_rpm] -> Mux6/1
  [CMP2_nM] -> Mux4/1
  Bus Selector6/1 -> Mux/4  "<aPres_S4>"
  [S5] -> Bus Selector7/1
  Mux/1 -> Out5/1
  Bus Selector5/3 -> Mux8/1  "<relHum_S3>"
  Bus Selector5/1 -> Mux/3  "<aPres_S3>"
  [S4] -> Bus Selector6/1
  Mux6/1 -> Out3/1
  [S3] -> Bus Selector5/1
  Bus Selector1/1 -> Mux2/1, EAT_Theo_Power/1(<mFlow_S1>), EAC_Theo_Power/1(<mFlow_S1>)  "<mFlow_S1>"
  Bus Selector7/1 -> Mux/5  "<aPres_S5>"
  Bus Selector8/1 -> EAT_Theo_Power/2(<aPres_S6>), Mux/6  "<aPres_S6>"
  [S1] -> Bus Selector1/1
  [Cathode_PresLvl] -> Mux/9
  Mux5/1 -> Out4/1
  Bus Selector6/3 -> Mux8/2  "<relHum_S4>"
  Bus Selector8/3 -> Mux8/4  "<relHum_S6>"
  [S6] -> Bus Selector8/1
  Bus Selector1/2 -> Mux/1, EAC_Theo_Power/2(<aPres_S1>)  "<aPres_S1>"
  [S2] -> Bus Selector4/1
  Mux4/1 -> Out2/1
  Mux1/1 -> Out7/1
  Mux8/1 -> Out8/1
  Bus Selector1/3 -> EAC_Theo_Power/4(<aTemp_S1>), Subsystem/1(<aTemp_S1>)  "<aTemp_S1>"
  Bus Selector4/2 -> Subsystem/2(<aTemp_S2>)  "<aTemp_S2>"
  Bus Selector5/2 -> Subsystem/3(<aTemp_S3>)  "<aTemp_S3>"
  Bus Selector6/2 -> Subsystem/4(<aTemp_S4>)  "<aTemp_S4>"
  Bus Selector7/2 -> Subsystem/5(<aTemp_S5>)  "<aTemp_S5>"
  Bus Selector8/2 -> EAT_Theo_Power/3(<aTemp_S6>), Subsystem/6(<aTemp_S6>)  "<aTemp_S6>"
  Bus Selector9/2 -> Subsystem/8(<aTemp_S7>)  "<aTemp_S8>"
  Subsystem/1(Out1) -> Mux1/1
  Subsystem/2(Out2) -> Mux1/2
  Subsystem/3(Out3) -> Mux1/3
  Subsystem/4(Out4) -> Mux1/4
  Subsystem/5(Out5) -> Mux1/5
  Subsystem/6(Out6) -> Mux1/6
  Subsystem/7(Out7) -> Mux1/7
  EAC_Theo_Power/1(Out1) -> Mux5/3
  EAT_Theo_Power/1(Out1) -> Mux5/4
  [S7] -> Bus Selector2/1
  Bus Selector2/2 -> Subsystem/7(In8)  "<aTemp_S7>"
  Subsystem/8(Out8) -> Mux1/8
  Bus Selector2/1 -> Mux/7  "<aPres_S7>"
  Bus Selector2/3 -> Mux8/5  "<relHum_S7>"
  [FCS_mdot_kgs_water] -> Mux2/2
  Mux2/1 -> <mFlow_S1>/1
  [Cathode_mFlow] -> Mux2/4
  [CWS_mdot_kgs_water] -> Mux2/3
  In1/1 -> Bus Selector/1
  Bus Selector/1 -> Mux/10  "<signal1>"
  Bus Selector/2 -> Mux1/9  "<signal2>"
  Bus Selector/5 -> Mux6/2  "<signal5>"
  Bus Selector/3 -> Mux5/5  "<signal3>"
  Bus Selector/4 -> Mux5/6  "<signal4>"

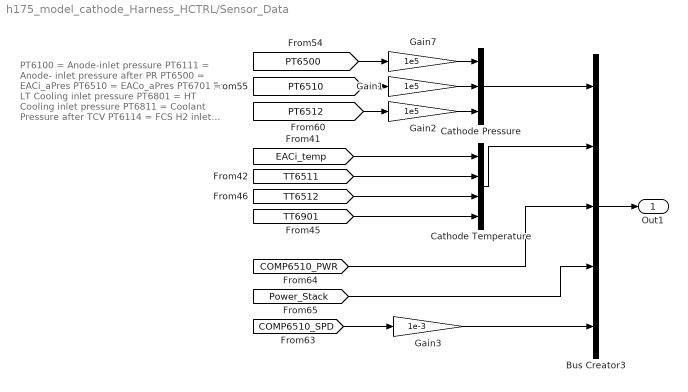
== system h175_model_cathode_Harness_HCTRL/Sensor_Data ==
  note: PT6100 = Anode-inlet pressure
      | PT6111 = Anode- inlet pressure after PR
      | PT6500 = EACi_aPres
      | PT6510 = EACo_aPres
      | PT6701 = LT Cooling inlet pressure
      | PT6801 = HT Cooling inlet pressure
      | PT6811 = Coolant Pressure after TCV
      | PT6114 = FCS H2 inlet pressure
      | PT6512 = FCS O2 inlet Pressure
      | PT6812 = FCS Coolant inlet pressure
      |
      | TT6100 = Anode- inlet Temperature
      | TT6111 = Anode- after Temperature
      | TT6500 = EACi_Temp
      | TT6510 = EACo_Temp
      | TT6701 = LT Cooling inlet Temperature
      | TT6801 = HT Cooling inlet Temperature
      | TT6811 = Coolant Temperature after TCV
      | TT6114 = FCS H2 inlet Temperature
      | TT6512 = FCS O2 inlet Temperature
      | TT6812 = FCS Coolant inlet Temperature
  Bus Creator3 : BusCreator  Inputs=5
  Cathode Pressure : Mux  Inputs=3
  Cathode Temperature : Mux
  Gain1 : Gain  Gain=1e5
  Gain2 : Gain  Gain=1e5
  Gain3 : Gain  Gain=1e-3
  Gain7 : Gain  Gain=1e5
  Out1 : Outport
  wires:
  Gain7/1 -> Cathode Pressure/1
  [PT6500] -> Gain7/1
  [PT6510] -> Gain1/1
  [COMP6510_SPD] -> Gain3/1
  [Power_Stack] -> Bus Creator3/4
  [COMP6510_PWR] -> Bus Creator3/3
  [PT6512] -> Gain2/1
  Gain1/1 -> Cathode Pressure/2
  [EACi_temp] -> Cathode Temperature/1
  [TT6511] -> Cathode Temperature/2
  Gain2/1 -> Cathode Pressure/3
  [TT6901] -> Cathode Temperature/4
  [TT6512] -> Cathode Temperature/3
  Cathode Pressure/1 -> Bus Creator3/1
  Cathode Temperature/1 -> Bus Creator3/2
  Bus Creator3/1 -> Out1/1
  Gain3/1 -> Bus Creator3/5

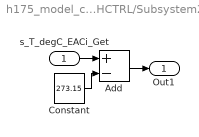
== system h175_model_cathode_Harness_HCTRL/Subsystem2 ==
  s_T_degC_EACi_Get : Inport
  Add : Sum  Inputs=+-
  Constant : Constant  Value=273.15
  Out1 : Outport
  wires:
  Add/1 -> Out1/1
  Constant/1 -> Add/2
  s_T_degC_EACi_Get/1 -> Add/1

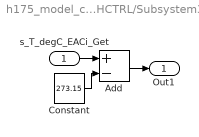
== system h175_model_cathode_Harness_HCTRL/Subsystem3 ==
  s_T_degC_EACi_Get : Inport
  Add : Sum  Inputs=+-
  Constant : Constant  Value=273.15
  Out1 : Outport
  wires:
  s_T_degC_EACi_Get/1 -> Add/1
  Constant/1 -> Add/2
  Add/1 -> Out1/1

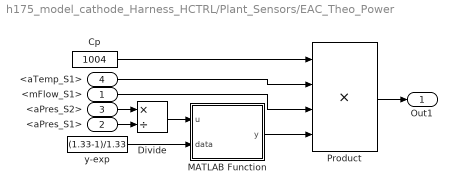
== system h175_model_cathode_Harness_HCTRL/Plant_Sensors/EAC_Theo_Power ==
  <mFlow_S1> : Inport
  <aPres_S1> : Inport  Port=2
  <aPres_S2> : Inport  Port=3
  <aTemp_S1> : Inport  Port=4
  Cp : Constant  Value=1004
  Divide : Product  Inputs=*/
  MATLAB Function : MATLAB Function  TreatAsAtomicUnit=on
  Product : Product  Inputs=4
  y-exp : Constant  Value=(1.33-1)/1.33
  Out1 : Outport
  wires:
  Cp/1 -> Product/1
  <aTemp_S1>/1 -> Product/2
  <aPres_S1>/1 -> Divide/2
  Product/1 -> Out1/1
  <aPres_S2>/1 -> Divide/1
  MATLAB Function/1(y) -> Product/4
  y-exp/1 -> MATLAB Function/2(data)
  Divide/1 -> MATLAB Function/1(u)
  <mFlow_S1>/1 -> Product/3

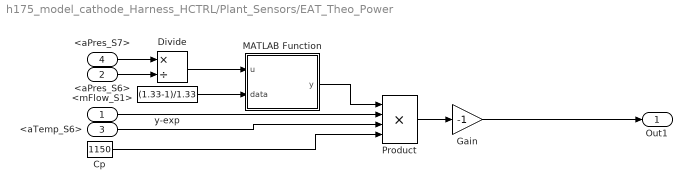
== system h175_model_cathode_Harness_HCTRL/Plant_Sensors/EAT_Theo_Power ==
  <mFlow_S1> : Inport
  <aPres_S6> : Inport  Port=2
  <aTemp_S6> : Inport  Port=3
  <aPres_S7> : Inport  Port=4
  Cp : Constant  Value=1150
  Divide : Product  Inputs=*/
  Gain : Gain  Gain=-1
  MATLAB Function : MATLAB Function  TreatAsAtomicUnit=on
  Product : Product  Inputs=4
  y-exp : Constant  Value=(1.33-1)/1.33
  Out1 : Outport
  wires:
  y-exp/1 -> MATLAB Function/2(data)
  <aPres_S7>/1 -> Divide/1
  Cp/1 -> Product/4
  Divide/1 -> MATLAB Function/1(u)
  Product/1 -> Gain/1
  <mFlow_S1>/1 -> Product/2
  MATLAB Function/1(y) -> Product/1
  <aTemp_S6>/1 -> Product/3
  <aPres_S6>/1 -> Divide/2
  Gain/1 -> Out1/1

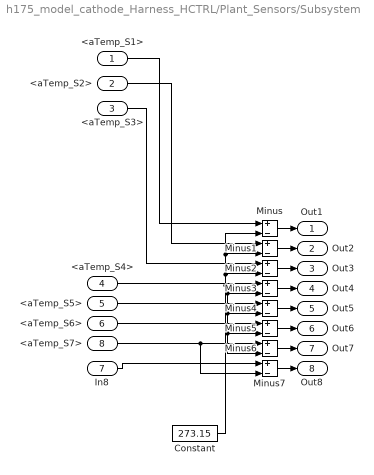
== system h175_model_cathode_Harness_HCTRL/Plant_Sensors/Subsystem ==
  <aTemp_S1> : Inport
  <aTemp_S2> : Inport  Port=2
  <aTemp_S3> : Inport  Port=3
  <aTemp_S4> : Inport  Port=4
  <aTemp_S5> : Inport  Port=5
  <aTemp_S6> : Inport  Port=6
  In8 : Inport  Port=7
  <aTemp_S7> : Inport  Port=8
  Constant : Constant  Value=273.15
  Minus{,1..7} (8 alike) : Sum  Inputs=+-
  Out1 : Outport
  Out2 : Outport  Port=2
  Out3 : Outport  Port=3
  Out4 : Outport  Port=4
  Out5 : Outport  Port=5
  Out6 : Outport  Port=6
  Out7 : Outport  Port=7
  Out8 : Outport  Port=8
  wires:
  Minus4/1 -> Out5/1
  Constant/1 -> Minus6/2, Minus5/2, Minus4/2, Minus3/2, Minus2/2, Minus1/2, Minus/2
  Minus2/1 -> Out3/1
  <aTemp_S7>/1 -> Minus7/2, Minus6/1
  <aTemp_S4>/1 -> Minus3/1
  <aTemp_S1>/1 -> Minus/1
  Minus5/1 -> Out6/1
  Minus6/1 -> Out7/1
  <aTemp_S3>/1 -> Minus2/1
  Minus/1 -> Out1/1
  <aTemp_S5>/1 -> Minus4/1
  Minus3/1 -> Out4/1
  Minus1/1 -> Out2/1
  <aTemp_S6>/1 -> Minus5/1
  <aTemp_S2>/1 -> Minus1/1
  In8/1 -> Minus7/1
  Minus7/1 -> Out8/1

== matlab function h175_model_cathode_Harness_HCTRL/Plant_Sensors/EAT_Theo_Power/MATLAB Function ==
  data: u input; y output; data input
function y = fcn(u, data)

y = (u^data)-1;

== matlab function h175_model_cathode_Harness_HCTRL/Plant_Sensors/EAC_Theo_Power/MATLAB Function ==
  data: u input; y output; data input
function y = fcn(u, data)

y = (u^data)-1;
